simulink model "circuitTestSimulink_MDKTemplate_NoDev_3DThermal"  (R2024b)
settings: Solver=VariableStepAuto  StartTime=0.0  StopTime=150  FixedStep=timestep  MaxStep=0.005  RelTol=1e-3  AbsTol=1e-3
undefined symbols (not defined in the file or in its folder): FMIKit
libraries: fl_lib x12, nesl_utility x9, ee_lib x2
settings Model: PacingRate=1000  Creator=ezzbj2  LastModifiedBy=Bawar
settings SolverCC: InitialStep=0.001  ZeroCrossControl=DisableAll  ZeroCrossAlgorithm=Adaptive
settings RTWCC: GPUComputeCapability=3.5

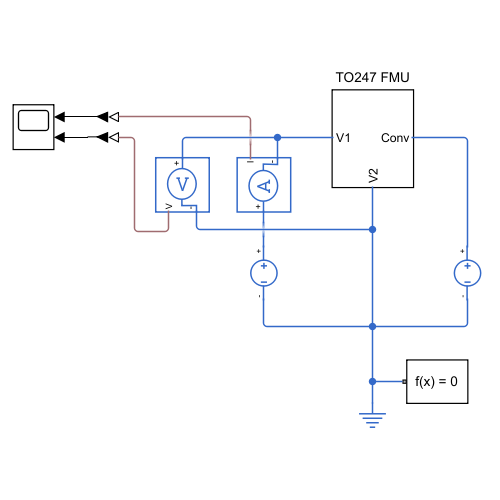
[thumbnail: Simulink's stored preview of the top-level diagram]
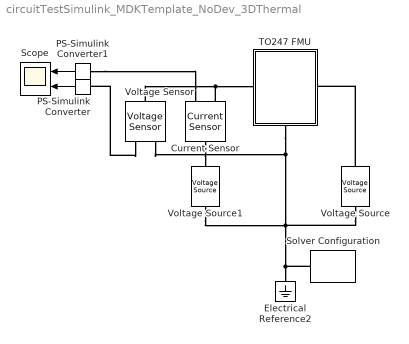
== system circuitTestSimulink_MDKTemplate_NoDev_3DThermal ==
  Current Sensor : fl_lib/Electrical/Electrical Sensors/Current Sensor
  Electrical Reference2 : fl_lib/Electrical/Electrical Elements/Electrical Reference
  PS-Simulink Converter : nesl_utility/PS-Simulink Converter  PhysicalDomain=network_engine_domain  SubClassName=ps_output  LeftPortType=input  RightPortType=output  PseudoPeriodic=off  Frequencies=[]  VectorFormat=inherit  Unit=inherit  AffineConversion=off
  PS-Simulink Converter1 : nesl_utility/PS-Simulink Converter  PhysicalDomain=network_engine_domain  SubClassName=ps_output  LeftPortType=input  RightPortType=output  PseudoPeriodic=off  Frequencies=[]  VectorFormat=inherit  Unit=inherit  AffineConversion=off
  Scope : Scope  NumInputPorts=2
  Solver Configuration : nesl_utility/Solver Configuration  PhysicalDomain=network_engine_domain  SubClassName=solver  LeftPortType=input  RightPortType=generic  Tones=[]  Harmonics=[]  SimulateNoise=off  Profile=off  UseLocalSampling=off  EnableSwitchedLinearOptims=on  FrequencyDomain=off  UseCCode=off  RelTol=0.001  AbsTol=0.001  MinStep=1e-09  ToWorkspace=off  RevertToSquareIcSolve=off  NumHomotopyIterations=100  PhasorMode=off  PhasorModeNumHarmonics=1  ConsistencySolver=NEWTON_XTOL_AFTER_FTOL  IndexReductionMethod=None  DoDC=off  ResidualTolerance=1e-09  ConsistencyTolSource=GLOBAL  ConsistencyAbsTol=0.001  ConsistencyRelTol=0.001  ConsistencyTolFactor=0.001  UseLocalSolver=off  LocalSolverChoice=NE_BACKWARD_EULER_ADVANCER  ResolveIndetEquations=on  FunctionEvalNumThread=1  LocalSolverSampleTime=1e-3  DoFixedCost=off  MaxNonlinIter=30  MaxModeIter=2  ComputeImpulses=on  ImpulseIterations=2  LinearAlgebra=auto  LinearAlgebraNumThread=0  EquationFormulation=NE_TIME_EF  DelaysMemoryBudget=1024  AutomaticFiltering=off  FilteringTimeConstant=0.001  PartitionStorageMethod=EXHAUSTIVE  PartitionMemoryBudget=1024  PartitionMethod=ROBUST  MultibodyUseLocalSolver=off  MultibodyLocalSolverChoice=ODE1  MultibodyLocalSolverSampleTime=0.001
  TO247 FMU : Subsystem
      settings: PortSchema="{\"entries\":[{\"content\":{\"sides\":[{\"content\":{\"connectorIds\":[\"LConn1\"]},\"type\":\"ConnectorPlacement.EquallySpacedRectSide\",\"uuid\":\"1a7c621a-b2c4-44d6-8085-8acdfe65af3e\"},{\"content\":{\"connectorIds\":[\"RConn1\"],\"side\":\"RIGHT\"},\"type\":\"ConnectorPlacement.EquallySpacedRectSide\",\"uuid\":\"009b5a79-97ab-42cc-83a0-e109b769c9f7\"},{\"content\":{\"side\":\"TOP\"},\"type\":\"ConnectorPlacement.EquallySpacedRectSide\",\"uuid\":\"b2698f3e-d975-41db-922f-800e4c377170\"},{\"content\":{\"connectorIds\":[\"RConn2\"],\"side\":\"BOTTOM\"},\"type\":\"ConnectorPlacement.EquallySpacedRectSide\",\"uuid\":\"c87b7d4f-b69b-4cab-ae10-03d23c792008\"}]},\"type\":\"ConnectorPlacement.EquallySpacedConnector\",\"uuid\":\"776127ee-5564-4d8f-a192-88fd759918ca\"}],\"packageUris\":[\"http://schema.mathworks.com/mf0/Connector/R2020b\"],\"version\":\"1.0\"}"
  Voltage Sensor : fl_lib/Electrical/Electrical Sensors/Voltage Sensor
  Voltage Source : ee_lib/Sources/Voltage Source  dc_voltage=0 V  ac_voltage=0 V  ac_shift=0 rad  ac_frequency=60 Hz  noise_mode=ee.enum.sources.noise.Disabled  PSD=0 V^2/Hz  sample_time=1e-3 s  repeatability=ee.enum.sources.repeatability.NotRepeatable  user_seed=0  auto_seed=3890346746  i_specify=off  i_priority=None  i=0 A  i_nominal_specify=off  i_nominal_value=1  i_nominal_unit=A  v_specify=off  v_priority=None  v=0 V  v_nominal_specify=off  v_nominal_value=1  v_nominal_unit=V
  Voltage Source1 : ee_lib/Sources/Voltage Source  dc_voltage=1 V  ac_voltage=0 V  ac_shift=0 rad  ac_frequency=60 Hz  noise_mode=ee.enum.sources.noise.Disabled  PSD=0 V^2/Hz  sample_time=1e-3 s  repeatability=ee.enum.sources.repeatability.NotRepeatable  user_seed=0  auto_seed=3499211588  i_specify=off  i_priority=None  i=0 A  i_nominal_specify=off  i_nominal_value=1  i_nominal_unit=A  v_specify=off  v_priority=None  v=0 V  v_nominal_specify=off  v_nominal_value=1  v_nominal_unit=V
  wires:
  PS-Simulink Converter/1 -> Scope/2
  PS-Simulink Converter1/1 -> Scope/1
  connections:
  Voltage Sensor/RConn2 -- TO247 FMU/RConn2 -- Voltage Source1/RConn1 -- Voltage Source/RConn1 -- Solver Configuration/RConn1 -- Electrical Reference2/LConn1
  Voltage Source/LConn1 -- TO247 FMU/RConn1
  Voltage Sensor/LConn1 -- Current Sensor/RConn2 -- TO247 FMU/LConn1
  Voltage Sensor/RConn1 -- PS-Simulink Converter/LConn1
  PS-Simulink Converter1/LConn1 -- Current Sensor/RConn1
  Current Sensor/LConn1 -- Voltage Source1/LConn1

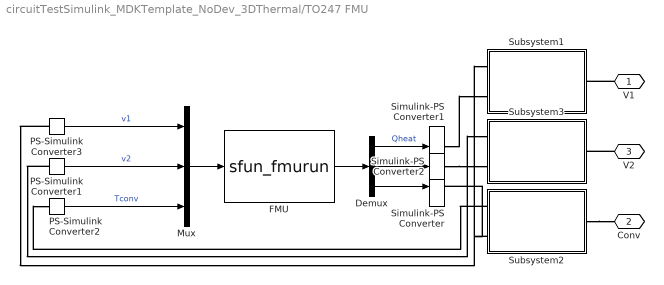
== system circuitTestSimulink_MDKTemplate_NoDev_3DThermal/TO247 FMU ==
  Demux : Demux  Outputs=3
  FMU : S-Function  LoadFcn=FMIKit.setSFunctionParameters(gcb)  FunctionName=sfun_fmurun  Parameters=3.0 0 '{D773325B-AB94-4630-BF85-643EB24FCB82}' 'MDKCircuit_NoDev_3DThermal' FMIKit.getUnzipDirectory(gcb) 1 1 0 'circuitTestSimulink_MDKTemplate_NoDev_3DThermal_TO247_FMU_FMU.txt' FMIKit.getSolverRelativeTolerance(bdroot(gcb)) -1 0 30 0 0 [3] [0.0] [2] [9] [3] [2] [10]  SFunctionDeploymentMode=off  EnableBusSupport=off
      settings: DeleteFcn=FMIKit.closeBlockDialog(gcbh)  ModelCloseFcn=FMIKit.closeBlockDialog(gcbh)  DestroyFcn=FMIKit.closeBlockDialog(gcbh)  OpenFcn=FMIKit.showBlockDialog(gcbh);  CloseFcn=FMIKit.closeBlockDialog(gcbh)  ParentCloseFcn=FMIKit.closeBlockDialog(gcbh)
      mask Help: eval('FMIKit.showBlockDialogHelp();')
      mask Display:
      | port_label('input', 1, 'u');
      | port_label('output', 1, 'y');
  Mux : Mux  Inputs=3
  PS-Simulink Converter1 : nesl_utility/PS-Simulink Converter  PhysicalDomain=network_engine_domain  SubClassName=ps_output  LeftPortType=input  RightPortType=output  PseudoPeriodic=off  Frequencies=[]  VectorFormat=inherit  Unit=inherit  AffineConversion=off
  PS-Simulink Converter2 : nesl_utility/PS-Simulink Converter  PhysicalDomain=network_engine_domain  SubClassName=ps_output  LeftPortType=input  RightPortType=output  PseudoPeriodic=off  Frequencies=[]  VectorFormat=inherit  Unit=inherit  AffineConversion=off
  PS-Simulink Converter3 : nesl_utility/PS-Simulink Converter  PhysicalDomain=network_engine_domain  SubClassName=ps_output  LeftPortType=input  RightPortType=output  PseudoPeriodic=off  Frequencies=[]  VectorFormat=inherit  Unit=inherit  AffineConversion=off
  Simulink-PS Converter : nesl_utility/Simulink-PS Converter  PhysicalDomain=network_engine_domain  SubClassName=ps_input  LeftPortType=input  RightPortType=output  PseudoPeriodic=off  Frequencies=[]  NoiseDistribution=none  NoiseParameters=[]  Unit=1  AffineConversion=off  FilteringAndDerivatives=zero  SimscapeFilterOrder=1  InputFilterTimeConstant=1e-9  UdotUserProvided=1
  Simulink-PS Converter1 : nesl_utility/Simulink-PS Converter  PhysicalDomain=network_engine_domain  SubClassName=ps_input  LeftPortType=input  RightPortType=output  PseudoPeriodic=off  Frequencies=[]  NoiseDistribution=none  NoiseParameters=[]  Unit=1  AffineConversion=off  FilteringAndDerivatives=zero  SimscapeFilterOrder=1  InputFilterTimeConstant=1e-9  UdotUserProvided=1
  Simulink-PS Converter2 : nesl_utility/Simulink-PS Converter  PhysicalDomain=network_engine_domain  SubClassName=ps_input  LeftPortType=input  RightPortType=output  PseudoPeriodic=off  Frequencies=[]  NoiseDistribution=none  NoiseParameters=[]  Unit=1  AffineConversion=off  FilteringAndDerivatives=zero  SimscapeFilterOrder=1  InputFilterTimeConstant=1e-9  UdotUserProvided=1
  Subsystem1 : Subsystem
  Subsystem2 : Subsystem
  Subsystem3 : Subsystem
  V1 : PMIOPort  Side=Left
  Conv : PMIOPort  Port=2  Side=Right
  V2 : PMIOPort  Port=3  Side=Right
  wires:
  PS-Simulink Converter3/1 -> Mux/1  "v1"
  Demux/1 -> Simulink-PS Converter1/1  "Qheat"
  FMU/1 -> Demux/1
  PS-Simulink Converter2/1 -> Mux/3  "Tconv"
  PS-Simulink Converter1/1 -> Mux/2  "v2"
  Demux/3 -> Simulink-PS Converter/1
  Demux/2 -> Simulink-PS Converter2/1
  Mux/1 -> FMU/1
  connections:
  Simulink-PS Converter1/RConn1 -- Subsystem1/LConn2
  PS-Simulink Converter3/LConn1 -- Subsystem1/LConn1
  Subsystem2/LConn2 -- Simulink-PS Converter/RConn1
  V1/RConn1 -- Subsystem1/RConn1
  Subsystem2/RConn1 -- Conv/RConn1
  Simulink-PS Converter2/RConn1 -- Subsystem3/LConn2
  PS-Simulink Converter1/LConn1 -- Subsystem3/LConn1
  V2/RConn1 -- Subsystem3/RConn1
  Subsystem2/LConn1 -- PS-Simulink Converter2/LConn1

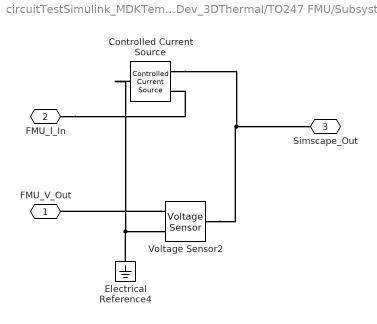
== system circuitTestSimulink_MDKTemplate_NoDev_3DThermal/TO247 FMU/Subsystem1 ==
  Controlled Current Source : fl_lib/Electrical/Electrical Sources/Controlled Current Source
  Electrical Reference4 : fl_lib/Electrical/Electrical Elements/Electrical Reference
  Voltage Sensor2 : fl_lib/Electrical/Electrical Sensors/Voltage Sensor
  FMU_V_Out : PMIOPort  Side=Left
  FMU_I_In : PMIOPort  Port=2  Side=Left
  Simscape_Out : PMIOPort  Port=3  Side=Right
  connections:
  Voltage Sensor2/RConn1 -- FMU_V_Out/RConn1
  FMU_I_In/RConn1 -- Controlled Current Source/RConn1
  Electrical Reference4/LConn1 -- Controlled Current Source/LConn1 -- Voltage Sensor2/RConn2
  Voltage Sensor2/LConn1 -- Controlled Current Source/RConn2 -- Simscape_Out/RConn1

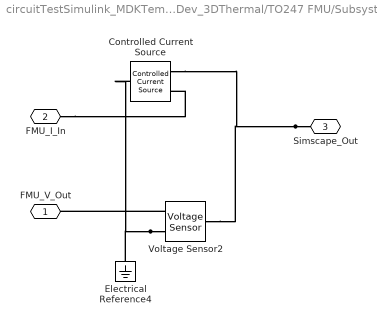
== system circuitTestSimulink_MDKTemplate_NoDev_3DThermal/TO247 FMU/Subsystem2 ==
  Controlled Current Source : fl_lib/Electrical/Electrical Sources/Controlled Current Source
  Electrical Reference4 : fl_lib/Electrical/Electrical Elements/Electrical Reference
  Voltage Sensor2 : fl_lib/Electrical/Electrical Sensors/Voltage Sensor
  FMU_V_Out : PMIOPort  Side=Left
  FMU_I_In : PMIOPort  Port=2  Side=Left
  Simscape_Out : PMIOPort  Port=3  Side=Right
  connections:
  Voltage Sensor2/RConn1 -- FMU_V_Out/RConn1
  FMU_I_In/RConn1 -- Controlled Current Source/RConn1
  Voltage Sensor2/RConn2 -- Electrical Reference4/LConn1 -- Controlled Current Source/LConn1
  Simscape_Out/RConn1 -- Voltage Sensor2/LConn1 -- Controlled Current Source/RConn2

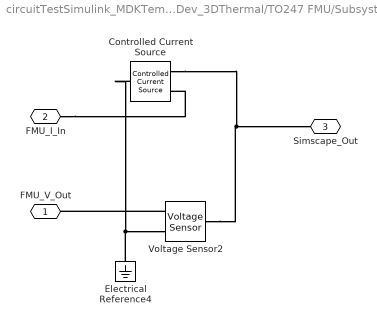
== system circuitTestSimulink_MDKTemplate_NoDev_3DThermal/TO247 FMU/Subsystem3 ==
  Controlled Current Source : fl_lib/Electrical/Electrical Sources/Controlled Current Source
  Electrical Reference4 : fl_lib/Electrical/Electrical Elements/Electrical Reference
  Voltage Sensor2 : fl_lib/Electrical/Electrical Sensors/Voltage Sensor
  FMU_V_Out : PMIOPort  Side=Left
  FMU_I_In : PMIOPort  Port=2  Side=Left
  Simscape_Out : PMIOPort  Port=3  Side=Right
  connections:
  Voltage Sensor2/RConn1 -- FMU_V_Out/RConn1
  FMU_I_In/RConn1 -- Controlled Current Source/RConn1
  Electrical Reference4/LConn1 -- Controlled Current Source/LConn1 -- Voltage Sensor2/RConn2
  Voltage Sensor2/LConn1 -- Controlled Current Source/RConn2 -- Simscape_Out/RConn1
